simulink library "observer"  (R2024a)
settings: Solver=VariableStepAuto  StartTime=0.0  StopTime=10.0  RelTol=1e-3
undefined symbols (not defined in the file): A, B, C, D, x_eq
settings Model: Creator=Bocchio  LastModifiedBy=Bocchio

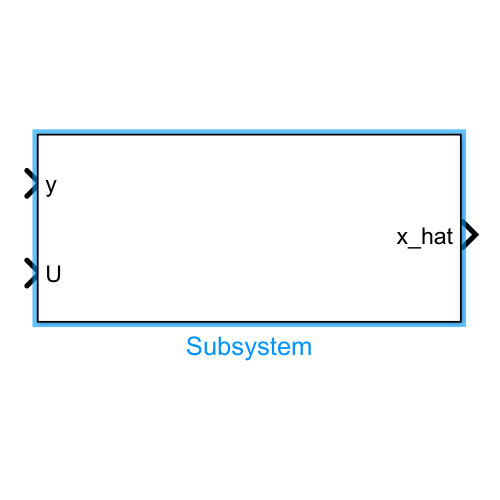
[thumbnail: Simulink's stored preview of the top-level diagram]
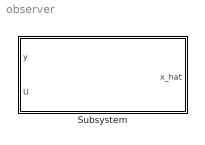
== system observer ==
  Subsystem : Subsystem  mask{L=0}
      mask DialogControl DescGroupVar Prompt: Generic Observer
      mask DialogControl DescTextVar Prompt: This component implements an observer of the type (A-L*C)

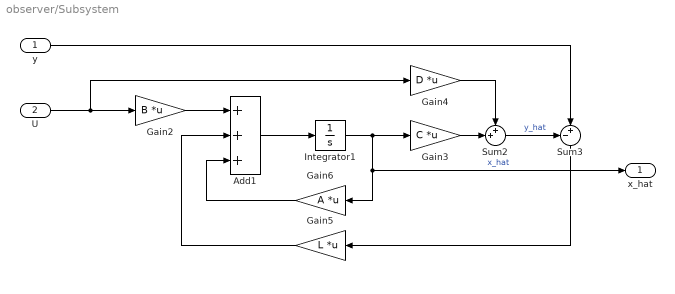
== system observer/Subsystem ==
  y : Inport
  U : Inport  Port=2
  Add1 : Sum  Inputs=+++
  Gain2 : Gain  Gain=B  Multiplication=Matrix(K*u)
  Gain3 : Gain  Gain=C  Multiplication=Matrix(K*u)
  Gain4 : Gain  Gain=D  Multiplication=Matrix(K*u)
  Gain5 : Gain  Gain=L  Multiplication=Matrix(K*u)
  Gain6 : Gain  Gain=A  Multiplication=Matrix(K*u)
  Integrator1 : Integrator  InitialCondition=x_eq
  Sum2 : Sum  Inputs=++|
  Sum3 : Sum  Inputs=-+|
  x_hat : Outport
  wires:
  Gain4/1 -> Sum2/1
  Sum3/1 -> Gain5/1
  Gain2/1 -> Add1/1
  Sum2/1 -> Sum3/1  "y_hat"
  Gain5/1 -> Add1/2
  Gain6/1 -> Add1/3
  U/1 -> Gain4/1, Gain2/1
  Add1/1 -> Integrator1/1
  Gain3/1 -> Sum2/2
  Integrator1/1 -> x_hat/1, Gain6/1, Gain3/1  "x_hat"
  y/1 -> Sum3/2
